simulink model "SINS"  (R2025b)
settings: Solver=VariableStepAuto  StartTime=0.0  StopTime=30  RelTol=1e-3
values from neighbouring files (symbols this model uses):
  dt_gps = 0.1    [init_sim.m]
  Empuje_Max = 8000    [init_sim.m]
  gps_pos_noise = 2.0    (= 2)    [init_sim.m]
  I_tensor = diag([Ixx, Iyy, Izz])    [init_sim.m]
  imu_accel_bias = 1 * 9.81 / 1000    (= 0.00981)    [init_sim.m]
  imu_accel_noise = 0.005    [init_sim.m]
  imu_gyro_bias = (1 / 3600) * (pi / 180)    (= 4.8481368111e-06)    [init_sim.m]
  imu_gyro_noise = 0.001    [init_sim.m]
  lat_0 = 40.4168    [init_sim.m]
  lon_0 = -3.7038    [init_sim.m]
  masa_0 = 150    [init_sim.m]
  t_burn = 10    [init_sim.m]
libraries: aerolibanim x1, aerolibnav x1
settings Model: Creator=Pc  LastModifiedBy=Pc

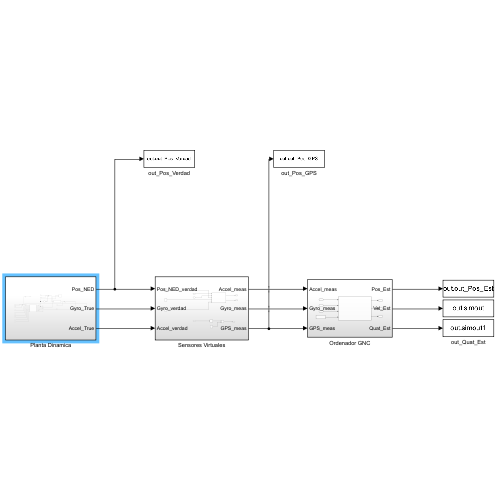
[thumbnail: Simulink's stored preview of the top-level diagram]
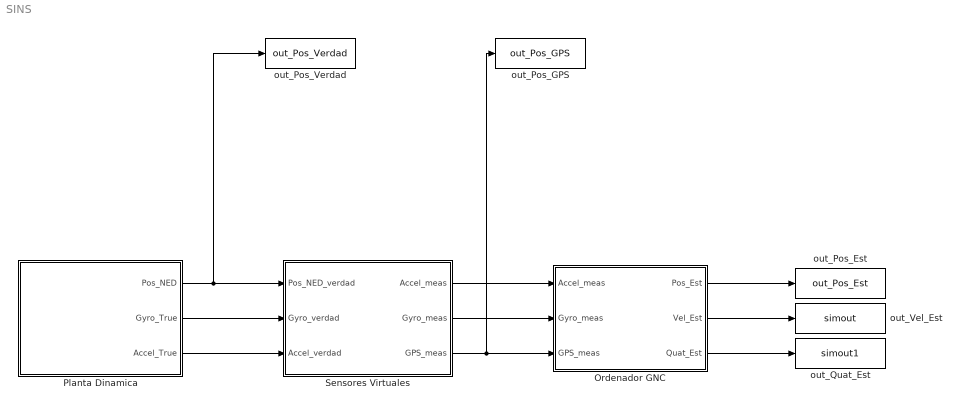
== system SINS ==
  Ordenador GNC : Subsystem
  Planta Dinamica : Subsystem
  Sensores Virtuales : Subsystem
  out_Pos_Est : ToWorkspace  VariableName=out_Pos_Est  SaveFormat=Timeseries  SampleTime=-1
  out_Pos_GPS : ToWorkspace  VariableName=out_Pos_GPS  SaveFormat=Timeseries  SampleTime=-1
  out_Pos_Verdad : ToWorkspace  VariableName=out_Pos_Verdad  SaveFormat=Timeseries  SampleTime=-1
  out_Quat_Est : ToWorkspace  VariableName=simout1  SaveFormat=Timeseries  SampleTime=-1
  out_Vel_Est : ToWorkspace  VariableName=simout  SaveFormat=Timeseries  SampleTime=-1
  wires:
  Planta Dinamica/2(Gyro_True) -> Sensores Virtuales/2(Gyro_verdad)
  Planta Dinamica/1(Pos_NED) -> out_Pos_Verdad/1, Sensores Virtuales/1(Pos_NED_verdad)
  Planta Dinamica/3(Accel_True) -> Sensores Virtuales/3(Accel_verdad)
  Sensores Virtuales/3(GPS_meas) -> out_Pos_GPS/1, Ordenador GNC/3(GPS_meas)
  Ordenador GNC/1(Pos_Est) -> out_Pos_Est/1
  Ordenador GNC/2(Vel_Est) -> out_Vel_Est/1
  Ordenador GNC/3(Quat_Est) -> out_Quat_Est/1
  Sensores Virtuales/1(Accel_meas) -> Ordenador GNC/1(Accel_meas)
  Sensores Virtuales/2(Gyro_meas) -> Ordenador GNC/2(Gyro_meas)

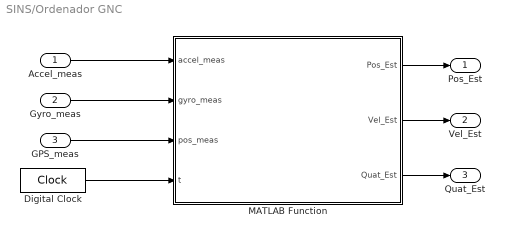
== system SINS/Ordenador GNC ==
  Accel_meas : Inport
  Gyro_meas : Inport  Port=2
  GPS_meas : Inport  Port=3
  Digital Clock : DigitalClock  SampleTime=0.005
  MATLAB Function : MATLAB Function  TreatAsAtomicUnit=on
  Pos_Est : Outport
  Vel_Est : Outport  Port=2
  Quat_Est : Outport  Port=3
  wires:
  Accel_meas/1 -> MATLAB Function/1(accel_meas)
  Gyro_meas/1 -> MATLAB Function/2(gyro_meas)
  GPS_meas/1 -> MATLAB Function/3(pos_meas)
  MATLAB Function/1(Pos_Est) -> Pos_Est/1
  MATLAB Function/2(Vel_Est) -> Vel_Est/1
  MATLAB Function/3(Quat_Est) -> Quat_Est/1
  Digital Clock/1 -> MATLAB Function/4(t)

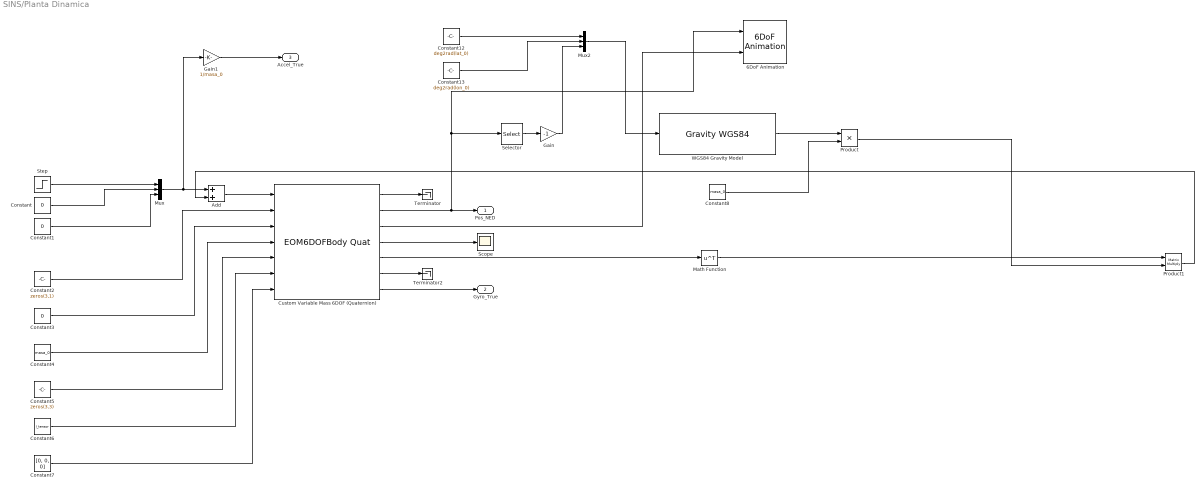
== system SINS/Planta Dinamica ==
  6DoF Animation : aerolibanim/6DoF Animation  u1=[0 4000 -2000 2000 -5000 -3000]  u2=0.1  u3=1.0  u4=[4000 0 -5000]  u5=Fixed position  u6=[2000 500 -3150]  u7=10  u8=on
  Add : Sum
  Constant : Constant  Value=0
  Constant1 : Constant  Value=0
  Constant12 : Constant  Value=deg2rad(lat_0)
  Constant13 : Constant  Value=deg2rad(lon_0)
  Constant2 : Constant  Value=zeros(3,1)
  Constant3 : Constant  Value=0
  Constant4 : Constant  Value=masa_0  VectorParams1D=off
  Constant5 : Constant  Value=zeros(3,3)
  Constant6 : Constant  Value=I_tensor
  Constant7 : Constant  Value=[0, 0, 0]
  Constant8 : Constant  Value=masa_0
  Custom Variable Mass 6DOF (Quaternion) : EOM6DOFBodyQuat  mtype=Custom Variable  xme_0=Pos_0_NED  Vm_0=V_body_0  eul_0=Euler_0  pm_0=omega_0  vre_flag=on
  Gain : Gain  Gain=-1
  Gain1 : Gain  Gain=1/masa_0
  Math Function : Math  Operator=transpose
  Mux : Mux  Inputs=3
  Mux2 : Mux  Inputs=3
  Product : Product
  Product1 : Product  Multiplication=Matrix(*)
  Scope : Scope
      settings: ActiveDisplayYMinimum=-0.34724020562630553  ActiveDisplayYMaximum=1.1361271675040994
  Selector : Selector  InputPortWidth=3  IndexOptions=Index vector (dialog)  Indices=3  OutputSizes=1
  Step : Step  Time=t_burn  Before=Empuje_Max  After=0  SampleTime=0
  Terminator : Terminator
  Terminator2 : Terminator
  "WGS84 Gravity Model  " : GravityWGS84
  Pos_NED : Outport
  Gyro_True : Outport  Port=2
  Accel_True : Outport  Port=3
  wires:
  Product/1 -> Product1/2
  Constant12/1 -> Mux2/1
  Mux2/1 -> "WGS84 Gravity Model  "/1
  Product1/1 -> Add/2
  "WGS84 Gravity Model  "/1 -> Product/1
  Constant3/1 -> Custom Variable Mass 6DOF (Quaternion)/3
  Constant/1 -> Mux/2
  Mux/1 -> Gain1/1, Add/1
  Selector/1 -> Gain/1
  Constant6/1 -> Custom Variable Mass 6DOF (Quaternion)/6
  Constant4/1 -> Custom Variable Mass 6DOF (Quaternion)/4
  Custom Variable Mass 6DOF (Quaternion)/1 -> Terminator/1
  Constant2/1 -> Custom Variable Mass 6DOF (Quaternion)/2
  Step/1 -> Mux/1
  Add/1 -> Custom Variable Mass 6DOF (Quaternion)/1
  Constant1/1 -> Mux/3
  Gain/1 -> Mux2/3
  Constant8/1 -> Product/2
  Constant5/1 -> Custom Variable Mass 6DOF (Quaternion)/5
  Custom Variable Mass 6DOF (Quaternion)/7 -> Gyro_True/1
  Custom Variable Mass 6DOF (Quaternion)/4 -> Scope/1
  Custom Variable Mass 6DOF (Quaternion)/6 -> Terminator2/1
  Constant13/1 -> Mux2/2
  Constant7/1 -> Custom Variable Mass 6DOF (Quaternion)/7
  Custom Variable Mass 6DOF (Quaternion)/2 -> Selector/1, 6DoF Animation/1, Pos_NED/1
  Gain1/1 -> Accel_True/1
  Custom Variable Mass 6DOF (Quaternion)/3 -> 6DoF Animation/2
  Custom Variable Mass 6DOF (Quaternion)/5 -> Math Function/1
  Math Function/1 -> Product1/1

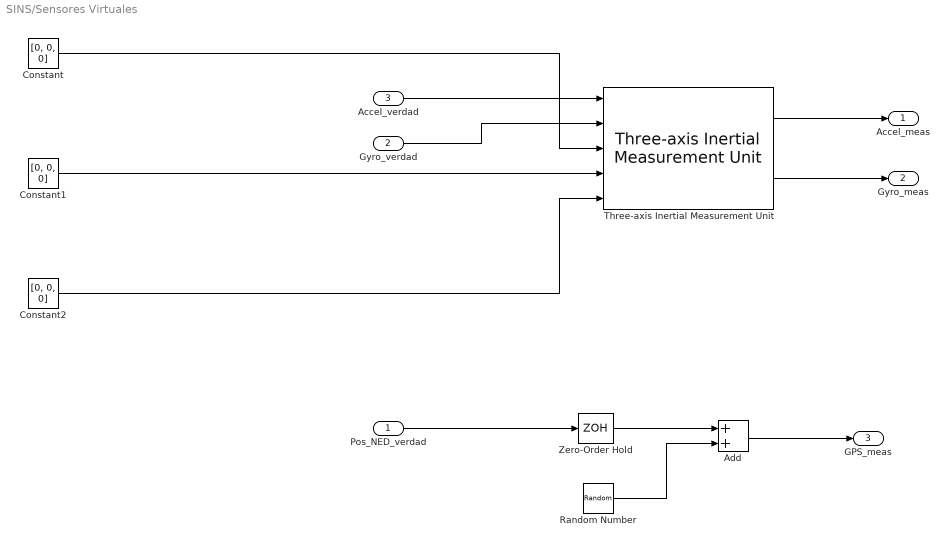
== system SINS/Sensores Virtuales ==
  Pos_NED_verdad : Inport
  Gyro_verdad : Inport  Port=2
  Accel_verdad : Inport  Port=3
  Add : Sum
  Constant : Constant  Value=[0, 0, 0]
  Constant1 : Constant  Value=[0, 0, 0]
  Constant2 : Constant  Value=[0, 0, 0]
  Random Number : RandomNumber  Variance=[gps_pos_noise^2, gps_pos_noise^2, gps_pos_noise^2]  SampleTime=dt_gps
  Three-axis Inertial Measurement Unit : aerolibnav/Three-axis Inertial Measurement Unit  units=Metric (MKS)  imu=[0 0 0]  i_Ts=1/dt_gps  dtype_a=on  w_a=190  z_a=0.707  a_sf_cc=[1 0 0; 0 1 0; 0 0 1]  a_bias=[1, 1, 1]*imu_accel_bias  a_sat="[-inf  -inf  -inf  inf inf inf]"  dtype_g=on  w_g=190  z_g=0.707  g_sf_cc=[1 0 0; 0 1 0; 0 0 1]  g_bias=[1, 1, 1]*imu_gyro_bias  g_sens=[0 0 0]  g_sat="[-inf  -inf  -inf  inf inf inf]"  i_rand=on  i_seeds=[23093 23094 23095 23096 23097 23098]  i_pow=[imu_accel_noise, imu_accel_noise, imu_accel_noise, imu_gyro_noise, imu_gyro_noise, imu_gyro_noise]
  Zero-Order Hold : ZeroOrderHold  SampleTime=dt_gps
  Accel_meas : Outport
  Gyro_meas : Outport  Port=2
  GPS_meas : Outport  Port=3
  wires:
  Constant/1 -> Three-axis Inertial Measurement Unit/3
  Constant1/1 -> Three-axis Inertial Measurement Unit/4
  Constant2/1 -> Three-axis Inertial Measurement Unit/5
  Three-axis Inertial Measurement Unit/1 -> Accel_meas/1
  Three-axis Inertial Measurement Unit/2 -> Gyro_meas/1
  Pos_NED_verdad/1 -> Zero-Order Hold/1
  Zero-Order Hold/1 -> Add/1
  Random Number/1 -> Add/2
  Add/1 -> GPS_meas/1
  Accel_verdad/1 -> Three-axis Inertial Measurement Unit/1
  Gyro_verdad/1 -> Three-axis Inertial Measurement Unit/2

== matlab function SINS/Ordenador GNC/MATLAB Function ==
  settings: updateMethod=DISCRETE
  data: accel_meas input; Pos_Est output; gyro_meas input; pos_meas input; Vel_Est output; Quat_Est output; t input
function [Pos_Est, Vel_Est, Quat_Est] = Navegacion_ES_EKF(accel_meas, gyro_meas, pos_meas, t)
    Pos_Est  = zeros(3,1); Vel_Est  = zeros(3,1); Quat_Est = zeros(4,1);
    persistent EKF t_last_gps t_last_imu

    if isempty(EKF)
        % 1. ANCLAJE GEOGRÁFICO
        lat0 = 40.4168; lon0 = -3.7038; alt0 = 0.0;
        EKF = insfilterErrorState('IMUSampleRate', 200, 'ReferenceFrame', 'NED', ...
                                  'ReferenceLocation', [lat0, lon0, alt0]);
        
        % 2. ACTITUD
        yaw   = 45 * pi/180; 
        pitch = 20 * pi/180;
        roll  =  0 * pi/180;
        
        cy = cos(yaw/2); sy = sin(yaw/2);
        cp = cos(pitch/2); sp = sin(pitch/2);
        cr = cos(roll/2); sr = sin(roll/2);
        
        qw = cr*cp*cy + sr*sp*sy;
        qx = sr*cp*cy - cr*sp*sy;
        qy = cr*sp*cy + sr*cp*sy;
        qz = cr*cp*sy - sr*sp*cy;
        EKF.State(1:4) = [qw; qx; qy; qz]; 
        
        % 3. VELOCIDAD
        EKF.State(5:7) = [0; 0; 0];    
        
        % 4. POSICIÓN INICIAL
        EKF.State(8:10) = pos_meas(:)';         
        
        % Cronómetros iniciales para proteger las frecuencias
        t_last_gps = -0.1; 
        t_last_imu = -0.005;
    end

    % PROTECCIÓN CONTRA ACELERACIONES ABSURDAS
    accel_segura = accel_meas(:)';
    if norm(accel_segura) > 1000, accel_segura = [0, 0, -9.81]; end

    % FASE DE PREDICCIÓN (Blindada estrictamente a 200 Hz)
    
    if (t - t_last_imu) >= 0.0049
        predict(EKF, accel_segura, gyro_meas(:)'); 
        t_last_imu = t;
    end

    % FASE DE CORRECCIÓN (Sincronizada estrictamente a 10 Hz)
    if (t - t_last_gps) >= 0.099
        R_Tierra = 6371000; 
        lat0 = 40.4168; lon0 = -3.7038; alt0 = 0.0; 
        
        lat_gps = lat0 + (pos_meas(1) / R_Tierra) * (180/pi);
        lon_gps = lon0 + (pos_meas(2) / (R_Tierra * cos(lat0 * pi/180))) * (180/pi);
        alt_gps = alt0 - pos_meas(3); 
        
        fusegps(EKF, [lat_gps, lon_gps, alt_gps], diag([4.0, 4.0, 4.0]));
        t_last_gps = t; 
    end
    
    % EXTRACCIÓN
    [p, q, v] = pose(EKF);
    Pos_Est = p'; Vel_Est = v'; Quat_Est = compact(q)'; 
end
